simulink model "Sistema_Teste_Hugo_1"  (R2019a)
settings: Solver=ode23t  StartTime=0.0  StopTime=86400  MaxStep=6  RelTol=1e-3  EnableMultiTasking=on
InitFcn:
  | Dados_do_Sistema
undefined symbols (not defined in the file or in its folder): D1, Dados, Delta
libraries: powerlib x263, powerlib_meascontrol x79, dspsrcs4 x50
(part 1 of 5)
Description:
  | Copyright 2008-2014 The MathWorks, Inc.
settings Model: Creator=MathWorks  LastModifiedBy=hugo1
settings DataIOCC: LimitDataPoints=on  SaveFormat=Array  SignalLoggingSaveFormat=ModelDataLogs  SaveOutput=off  SaveTime=off  ReturnWorkspaceOutputs=off
settings OptimizationCC: ExpressionDepthLimit=2147483647  LifeSpan=inf
settings DebuggingCC: ReadBeforeWriteMsg=DisableAll  WriteAfterWriteMsg=DisableAll  WriteAfterReadMsg=DisableAll  UnderspecifiedInitializationDetection=Classic  MergeDetectMultiDrivingBlocksExec=none  SolverPrmCheckMsg=warning  ParameterPrecisionLossMsg=none  FcnCallInpInsideContextMsg=warning  UnconnectedInputMsg=none  UnconnectedOutputMsg=none  UnconnectedLineMsg=none  StateNameClashWarn=warning  SFUnexpectedBacktrackingDiag=warning  SFNoUnconditionalDefaultTransitionDiag=warning  SFExecutionAtInitializationDiag=none  ArithmeticOperatorsInVariantConditions=warning
settings HardwareCC: ProdBitPerPointer=32  ProdBitPerSizeT=32  ProdBitPerPtrDiffT=32  ProdLargestAtomicFloat=None  ProdIntDivRoundTo=Undefined  ProdEndianess=Unspecified  ProdWordSize=32  ProdHWDeviceType=32-bit Generic
settings ModelReferenceCC: PropagateSignalLabelsOutOfModel=off
settings SFSimCC: SimUseLocalCustomCode=off
settings RTWCC: RTWUseLocalCustomCode=off
settings CodeAppCC: StateflowObjectComments=on
settings GRTTargetCC: TargetLangStandard=C89/C90 (ANSI)  GeneratePreprocessorConditionals=Disable all  CombineOutputUpdateFcns=off  GRTInterface=on
settings ConfigComp: CovMetricSettings=dw  CovHtmlReporting=on  CovSaveCumulativeToWorkspaceVar=on  CovSaveSingleToWorkspaceVar=on  CovExternalEMLEnable=off  CovSFcnEnable=off
settings SimscapeCC: SimscapeNormalizeSystem=off

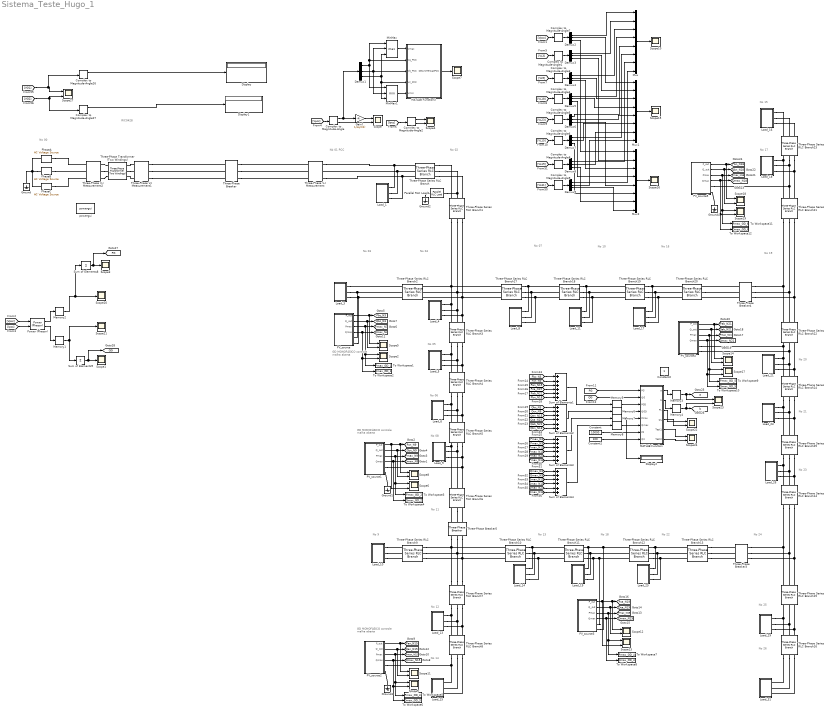
== system Sistema_Teste_Hugo_1 ==
  note: No 00
  note: RIC0428
  note: Nó 01 PCC
  note: No 02
  note: No 04
  note: No 03
  note: No 05
  note: No 06
  note: No 08
  note: No 11
  note: No 12
  note: No 14
  note: No 9
  note: No 13
  note: No 18
  note: No 22
  note: No 24
  note: No 25
  note: No 26
  note: No 20
  note: No 17
  note: No 15
  note: No 21
  note: No 23
  note: GD MONOFÁSICO
      | controle malha aberta
  note: GD MONOFÁSICO
      | controle malha aberta
  note: GD MONOFÁSICO
      | controle malha aberta
  note: No 07
  note: No 10
  note: No 16
  note: No 19
  Complex to Magnitude-Angle{,2,26..27} (4 alike) : ComplexToMagnitudeAngle
  Complex to Magnitude-Angle{1,3..9} (8 alike) : ComplexToMagnitudeAngle  Output=Magnitude
  Constant : Constant  Value=10000
  Constant1 : Constant  Value=100
  Constant2 : Constant
  Demux{1..9} (9 alike) : Demux  Outputs=3
  Display : Display
  Display1 : Display
  Display2 : Display
      settings: Decimation=3
  Gain1 : Gain  Gain=1/sqrt(2)
  Ground{,1..4} (5 alike) : powerlib/Elements/Ground  LConnTagsString=a
      settings: SourceProductName=Simscape Electrical
  Load_1 : Subsystem
  Load_10 : Subsystem
  Load_11 : Subsystem
  Load_13 : Subsystem
  Load_14 : Subsystem
  Load_15 : Subsystem
  Load_16 : Subsystem
  Load_17 : Subsystem
  Load_18 : Subsystem
  Load_19 : Subsystem
  Load_21 : Subsystem
  Load_23 : Subsystem
  Load_25 : Subsystem
  Load_26 : Subsystem
  Load_29 : Subsystem
  Load_3 : Subsystem
  Load_31 : Subsystem
  Load_4 : Subsystem
  Load_5 : Subsystem
  Load_6 : Subsystem
  Load_8 : Subsystem
  Load_9 : Subsystem
  MATLAB Function : MATLAB Function  TreatAsAtomicUnit=on
  MATLAB Function3 : MATLAB Function  TreatAsAtomicUnit=on
  Memory{1..8} (8 alike) : Memory
  MinMax : MinMax  Function=max  Inputs=3
  MinMax1 : MinMax  Inputs=3
  Mux : Mux  Inputs=8
  Mux1 : Mux  Inputs=8
  Mux2 : Mux  Inputs=8
  PV_source : Subsystem
  PV_source1 : Subsystem
  PV_source2 : Subsystem
  PV_source3 : Subsystem
  PV_source4 : Subsystem
  PV_source5 : Subsystem
  Parallel RLC Load1 : powerlib/Elements/Parallel RLC Load  LConnTagsString=a  RConnTagsString=__new0  NominalVoltage=127  NominalFrequency=60  ActivePower=100  InductivePower=40  CapacitivePower=0  Setx0=off  InitialVoltage=0  SetiL0=off  InitialCurrent=0  Measurements=None  LoadType=constant Z
      settings: AttributesFormatString=\n  SourceProductName=Simscape Electrical  SourceProductBaseCode=PS
  PhaseA : powerlib/Electrical Sources/AC Voltage Source  Amplitude=Dados.Tensao.va(1)  Phase=Dados.Tensao.va(2)  Frequency=Dados.Freq  SampleTime=0  Measurements=None  BusType=swing  Pref=10e3  Qref=0  Qmin=-inf  Qmax=+inf
      settings: SourceProductName=Simscape Electrical
  PhaseB : powerlib/Electrical Sources/AC Voltage Source  Amplitude=Dados.Tensao.vb(1)  Phase=Dados.Tensao.vb(2)  Frequency=Dados.Freq  SampleTime=0  Measurements=None  BusType=swing  Pref=10e3  Qref=0  Qmin=-inf  Qmax=+inf
      settings: SourceProductName=Simscape Electrical
  PhaseC : powerlib/Electrical Sources/AC Voltage Source  Amplitude=Dados.Tensao.vc(1)  Phase=Dados.Tensao.vc(2)  Frequency=Dados.Freq  SampleTime=0  Measurements=None  BusType=swing  Pref=10e3  Qref=0  Qmin=-inf  Qmax=+inf
      settings: SourceProductName=Simscape Electrical
  Power (Phasor) : powerlib_meascontrol/Measurements/Power (Phasor)
      settings: SourceProductName=Simscape Electrical  SourceProductBaseCode=PS
  Scope{,2,4..6,8..9,11..14,17..19,22..24,27} (18 alike) : Scope  NumInputPorts=2
  Scope{1,3,7,10,15..16,20..21} (8 alike) : Scope
  Sum of Elements{1..4} (4 alike) : Sum  Inputs=++++++
  Sum of Elements8 : Sum  Inputs=+
  Sum of Elements9 : Sum  Inputs=+
  Three-Phase Series RLC Branch : powerlib/Elements/Three-Phase Series RLC Branch  LConnTagsString=A|B|C  RConnTagsString=A|B|C  BranchType=RL  Resistance=Dados.Linha.Linha_01_02(1)  Inductance=Dados.Linha.Linha_01_02(2)  Capacitance=inf  Measurements=Branch currents
      settings: SourceProductName=Simscape Electrical
  Three-Phase Series RLC Branch1 : powerlib/Elements/Three-Phase Series RLC Branch  LConnTagsString=A|B|C  RConnTagsString=A|B|C  BranchType=RL  Resistance=Dados.Linha.Linha_02_04(1)  Inductance=Dados.Linha.Linha_02_04(2)  Capacitance=inf  Measurements=Branch currents
      settings: SourceProductName=Simscape Electrical
  Three-Phase Series RLC Branch10 : powerlib/Elements/Three-Phase Series RLC Branch  LConnTagsString=A|B|C  RConnTagsString=A|B|C  BranchType=RL  Resistance=Dados.Linha.Linha_11_13(1)  Inductance=Dados.Linha.Linha_11_13(2)  Capacitance=inf  Measurements=Branch currents
      settings: SourceProductName=Simscape Electrical
  Three-Phase Series RLC Branch11 : powerlib/Elements/Three-Phase Series RLC Branch  LConnTagsString=A|B|C  RConnTagsString=A|B|C  BranchType=RL  Resistance=Dados.Linha.Linha_13_18(1)  Inductance=Dados.Linha.Linha_13_18(2)  Capacitance=inf  Measurements=Branch currents
      settings: SourceProductName=Simscape Electrical
  Three-Phase Series RLC Branch12 : powerlib/Elements/Three-Phase Series RLC Branch  LConnTagsString=A|B|C  RConnTagsString=A|B|C  BranchType=RL  Resistance=Dados.Linha.Linha_18_22(1)  Inductance=Dados.Linha.Linha_18_22(2)  Capacitance=inf  Measurements=Branch currents
      settings: SourceProductName=Simscape Electrical
  Three-Phase Series RLC Branch13 : powerlib/Elements/Three-Phase Series RLC Branch  LConnTagsString=A|B|C  RConnTagsString=A|B|C  BranchType=RL  Resistance=Dados.Linha.Linha_22_24(1)  Inductance=Dados.Linha.Linha_22_24(2)  Capacitance=inf  Measurements=Branch currents
      settings: SourceProductName=Simscape Electrical
  Three-Phase Series RLC Branch14 : powerlib/Elements/Three-Phase Series RLC Branch  LConnTagsString=A|B|C  RConnTagsString=A|B|C  BranchType=RL  Resistance=Dados.Linha.Linha_24_23(1)  Inductance=Dados.Linha.Linha_24_23(2)  Capacitance=inf  Measurements=None
      settings: SourceProductName=Simscape Electrical
  Three-Phase Series RLC Branch15 : powerlib/Elements/Three-Phase Series RLC Branch  LConnTagsString=A|B|C  RConnTagsString=A|B|C  BranchType=RL  Resistance=Dados.Linha.Linha_24_25(1)  Inductance=Dados.Linha.Linha_24_25(2)  Capacitance=inf  Measurements=Branch currents
      settings: SourceProductName=Simscape Electrical
  Three-Phase Series RLC Branch16 : powerlib/Elements/Three-Phase Series RLC Branch  LConnTagsString=A|B|C  RConnTagsString=A|B|C  BranchType=RL  Resistance=Dados.Linha.Linha_25_26(1)  Inductance=Dados.Linha.Linha_25_26(2)  Capacitance=inf  Measurements=Branch currents
      settings: SourceProductName=Simscape Electrical
  Three-Phase Series RLC Branch17 : powerlib/Elements/Three-Phase Series RLC Branch  LConnTagsString=A|B|C  RConnTagsString=A|B|C  BranchType=RL  Resistance=Dados.Linha.Linha_07_04(1)  Inductance=Dados.Linha.Linha_07_04(2)  Capacitance=inf  Measurements=Branch currents
      settings: SourceProductName=Simscape Electrical
  Three-Phase Series RLC Branch18 : powerlib/Elements/Three-Phase Series RLC Branch  LConnTagsString=A|B|C  RConnTagsString=A|B|C  BranchType=RL  Resistance=Dados.Linha.Linha_10_07(1)  Inductance=Dados.Linha.Linha_10_07(2)  Capacitance=inf  Measurements=Branch currents
      settings: SourceProductName=Simscape Electrical
  Three-Phase Series RLC Branch19 : powerlib/Elements/Three-Phase Series RLC Branch  LConnTagsString=A|B|C  RConnTagsString=A|B|C  BranchType=RL  Resistance=Dados.Linha.Linha_16_10(1)  Inductance=Dados.Linha.Linha_16_10(2)  Capacitance=inf  Measurements=Branch currents
      settings: SourceProductName=Simscape Electrical
  Three-Phase Series RLC Branch2 : powerlib/Elements/Three-Phase Series RLC Branch  LConnTagsString=A|B|C  RConnTagsString=A|B|C  BranchType=RL  Resistance=Dados.Linha.Linha_04_03(1)  Inductance=Dados.Linha.Linha_04_03(2)  Capacitance=inf  Measurements=Branch currents
      settings: SourceProductName=Simscape Electrical
  Three-Phase Series RLC Branch20 : powerlib/Elements/Three-Phase Series RLC Branch  LConnTagsString=A|B|C  RConnTagsString=A|B|C  BranchType=RL  Resistance=Dados.Linha.Linha_19_16(1)  Inductance=Dados.Linha.Linha_19_16(2)  Capacitance=inf  Measurements=Branch currents
      settings: SourceProductName=Simscape Electrical
  Three-Phase Series RLC Branch21 : powerlib/Elements/Three-Phase Series RLC Branch  LConnTagsString=A|B|C  RConnTagsString=A|B|C  BranchType=RL  Resistance=Dados.Linha.Linha_19_17(1)  Inductance=Dados.Linha.Linha_19_17(2)  Capacitance=inf  Measurements=Branch currents
      settings: SourceProductName=Simscape Electrical
  Three-Phase Series RLC Branch22 : powerlib/Elements/Three-Phase Series RLC Branch  LConnTagsString=A|B|C  RConnTagsString=A|B|C  BranchType=RL  Resistance=Dados.Linha.Linha_20_19(1)  Inductance=Dados.Linha.Linha_20_19(2)  Capacitance=inf  Measurements=None
      settings: SourceProductName=Simscape Electrical
  Three-Phase Series RLC Branch23 : powerlib/Elements/Three-Phase Series RLC Branch  LConnTagsString=A|B|C  RConnTagsString=A|B|C  BranchType=RL  Resistance=Dados.Linha.Linha_17_15(1)  Inductance=Dados.Linha.Linha_17_15(2)  Capacitance=inf  Measurements=Branch currents
      settings: SourceProductName=Simscape Electrical
  Three-Phase Series RLC Branch24 : powerlib/Elements/Three-Phase Series RLC Branch  LConnTagsString=A|B|C  RConnTagsString=A|B|C  BranchType=RL  Resistance=Dados.Linha.Linha_21_20(1)  Inductance=Dados.Linha.Linha_21_20(2)  Capacitance=inf  Measurements=Branch currents
      settings: SourceProductName=Simscape Electrical
  Three-Phase Series RLC Branch25 : powerlib/Elements/Three-Phase Series RLC Branch  LConnTagsString=A|B|C  RConnTagsString=A|B|C  BranchType=RL  Resistance=Dados.Linha.Linha_23_21(1)  Inductance=Dados.Linha.Linha_23_21(2)  Capacitance=inf  Measurements=Branch currents
      settings: SourceProductName=Simscape Electrical
  Three-Phase Series RLC Branch3 : powerlib/Elements/Three-Phase Series RLC Branch  LConnTagsString=A|B|C  RConnTagsString=A|B|C  BranchType=RL  Resistance=Dados.Linha.Linha_04_05(1)  Inductance=Dados.Linha.Linha_04_05(2)  Capacitance=inf  Measurements=None
      settings: SourceProductName=Simscape Electrical
  Three-Phase Series RLC Branch4 : powerlib/Elements/Three-Phase Series RLC Branch  LConnTagsString=A|B|C  RConnTagsString=A|B|C  BranchType=RL  Resistance=Dados.Linha.Linha_05_06(1)  Inductance=Dados.Linha.Linha_05_06(2)  Capacitance=inf  Measurements=Branch currents
      settings: SourceProductName=Simscape Electrical
  Three-Phase Series RLC Branch5 : powerlib/Elements/Three-Phase Series RLC Branch  LConnTagsString=A|B|C  RConnTagsString=A|B|C  BranchType=RL  Resistance=Dados.Linha.Linha_06_08(1)  Inductance=Dados.Linha.Linha_06_08(2)  Capacitance=inf  Measurements=Branch currents
      settings: SourceProductName=Simscape Electrical
  Three-Phase Series RLC Branch6 : powerlib/Elements/Three-Phase Series RLC Branch  LConnTagsString=A|B|C  RConnTagsString=A|B|C  BranchType=RL  Resistance=Dados.Linha.Linha_08_11(1)  Inductance=Dados.Linha.Linha_08_11(2)  Capacitance=inf  Measurements=Branch currents
      settings: SourceProductName=Simscape Electrical
  Three-Phase Series RLC Branch7 : powerlib/Elements/Three-Phase Series RLC Branch  LConnTagsString=A|B|C  RConnTagsString=A|B|C  BranchType=RL  Resistance=Dados.Linha.Linha_11_12(1)  Inductance=Dados.Linha.Linha_11_12(2)  Capacitance=inf  Measurements=Branch currents
      settings: SourceProductName=Simscape Electrical
  Three-Phase Series RLC Branch8 : powerlib/Elements/Three-Phase Series RLC Branch  LConnTagsString=A|B|C  RConnTagsString=A|B|C  BranchType=RL  Resistance=Dados.Linha.Linha_12_14(1)  Inductance=Dados.Linha.Linha_12_14(2)  Capacitance=inf  Measurements=Branch currents
      settings: SourceProductName=Simscape Electrical
  Three-Phase Series RLC Branch9 : powerlib/Elements/Three-Phase Series RLC Branch  LConnTagsString=A|B|C  RConnTagsString=A|B|C  BranchType=RL  Resistance=Dados.Linha.Linha_11_09(1)  Inductance=Dados.Linha.Linha_11_09(2)  Capacitance=inf  Measurements=None
      settings: SourceProductName=Simscape Electrical
  Three-Phase Transformer (Two Windings) : powerlib/Elements/Three-Phase Transformer (Two Windings)  Winding1Connection=Delta (D1)  Winding2Connection=Yg  CoreType=Three single-phase transformers  SetSaturation=off  Hysteresis=off  DataFile='hysteresis'  SetInitialFlux=off  Measurements=None  UNITS=pu  NominalPower=[ 75e3 , 60 ]  Winding1=[ 13.8e3 , 0.0076 , 0.0157 ]  Winding2=[ 220 , 0.0076 , 0.0157 ]  Rm=227  Lm=32.59  L0=0.5  Saturation=[ 0,0 ; 0.0024,1.2 ; 1.0,1.52 ]  InitialFluxes=[ 0.8 , -0.8 , 0.7 ]  BreakLoop=off  DiscreteSolver=Trapezoidal iterative  DataType=off  TransfoNumber=1
      settings: SourceProductName=Simscape Electrical
  Three-Phase V-I Measurement : powerlib/Measurements/Three-Phase V-I Measurement  VoltageMeasurement=phase-to-ground  SetLabelV=on  LabelV=Vpcc  Vpu=off  VpuLL=off  CurrentMeasurement=yes  SetLabelI=on  LabelI=Ipcc  Ipu=off  Pbase=100e6  Vbase=500e3  OutputType=Complex  PhasorSimulation=on  PSBequivalent=0
      settings: SourceProductName=Simscape Electrical
  Three-Phase V-I Measurement1 : powerlib/Measurements/Three-Phase V-I Measurement  VoltageMeasurement=phase-to-phase  SetLabelV=on  LabelV=VG2  Vpu=off  VpuLL=off  CurrentMeasurement=no  SetLabelI=off  LabelI=IG  Ipu=off  Pbase=100e6  Vbase=500e3  OutputType=Complex  PhasorSimulation=on  PSBequivalent=0
      settings: SourceProductName=Simscape Electrical
  Three-Phase V-I Measurement2 : powerlib/Measurements/Three-Phase V-I Measurement  VoltageMeasurement=phase-to-phase  SetLabelV=on  LabelV=VG1  Vpu=off  VpuLL=off  CurrentMeasurement=no  SetLabelI=off  LabelI=IG  Ipu=off  Pbase=100e6  Vbase=500e3  OutputType=Complex  PhasorSimulation=on  PSBequivalent=0
      settings: SourceProductName=Simscape Electrical
  Three-Phase Breaker : powerlib/Elements/Three-Phase Breaker  InitialState=closed  SwitchA=on  SwitchB=on  SwitchC=on  SwitchTimes=[200000]  External=off  BreakerResistance=0.01  SnubberResistance=1e6  SnubberCapacitance=inf  Measurements=None
      settings: SourceProductName=Simscape Electrical
  Three-Phase Breaker3 : powerlib/Elements/Three-Phase Breaker  InitialState=closed  SwitchA=on  SwitchB=on  SwitchC=on  SwitchTimes=[864000]  External=off  BreakerResistance=0.01  SnubberResistance=1e6  SnubberCapacitance=inf  Measurements=None
      settings: SourceProductName=Simscape Electrical
  Three-Phase Breaker4 : powerlib/Elements/Three-Phase Breaker  InitialState=closed  SwitchA=on  SwitchB=on  SwitchC=on  SwitchTimes=[864000]  External=off  BreakerResistance=0.01  SnubberResistance=1e6  SnubberCapacitance=inf  Measurements=None
      settings: SourceProductName=Simscape Electrical
  Three-Phase Breaker5 : powerlib/Elements/Three-Phase Breaker  InitialState=closed  SwitchA=on  SwitchB=on  SwitchC=on  SwitchTimes=[864000]  External=off  BreakerResistance=0.01  SnubberResistance=1e6  SnubberCapacitance=inf  Measurements=None
      settings: SourceProductName=Simscape Electrical
  To Workspace1 : ToWorkspace  VariableName=Pmax_GD_1  SampleTime=-1
      settings: Save2DSignal=2-D array (concatenate along first dimension)
  To Workspace10 : ToWorkspace  VariableName=Qmax_GD_5  SampleTime=-1
      settings: Save2DSignal=2-D array (concatenate along first dimension)
  To Workspace11 : ToWorkspace  VariableName=Pmax_GD_6  SampleTime=-1
      settings: Save2DSignal=2-D array (concatenate along first dimension)
  To Workspace12 : ToWorkspace  VariableName=Qmax_GD_6  SampleTime=-1
      settings: Save2DSignal=2-D array (concatenate along first dimension)
  To Workspace2 : ToWorkspace  VariableName=Qmax_GD_1  SampleTime=-1
      settings: Save2DSignal=2-D array (concatenate along first dimension)
  To Workspace3 : ToWorkspace  VariableName=Pmax_GD_2  SampleTime=-1
      settings: Save2DSignal=2-D array (concatenate along first dimension)
  To Workspace4 : ToWorkspace  VariableName=Qmax_GD_2  SampleTime=-1
      settings: Save2DSignal=2-D array (concatenate along first dimension)
  To Workspace5 : ToWorkspace  VariableName=Pmax_GD_3  SampleTime=-1
      settings: Save2DSignal=2-D array (concatenate along first dimension)
  To Workspace6 : ToWorkspace  VariableName=Qmax_GD_3  SampleTime=-1
      settings: Save2DSignal=2-D array (concatenate along first dimension)
  To Workspace7 : ToWorkspace  VariableName=Pmax_GD_4  SampleTime=-1
      settings: Save2DSignal=2-D array (concatenate along first dimension)
  To Workspace8 : ToWorkspace  VariableName=Qmax_GD_4  SampleTime=-1
      settings: Save2DSignal=2-D array (concatenate along first dimension)
  To Workspace9 : ToWorkspace  VariableName=Pmax_GD_5  SampleTime=-1
      settings: Save2DSignal=2-D array (concatenate along first dimension)
  powergui : powerlib/powergui  Priority=1  SimulationMode=Phasor  SampleTime=50e-6  frequency=60  Iterations=50  frequencyindice=60  Pbase=100e6  ErrMax=1e-4  UnitsV=kV  UnitsW=MW  buscounter=0  FunctionMessages=off  echomessages=off  EnableUseOfTLC=off  CurrentSourceSwitches=off  DisableSnubberDevices=off  DisableRonSwitches=off  DisableVfSwitches=off  DisplayEquations=off  AutomaticDiscreteSolvers=off  SolverType=Tustin  Interpol=off  ExternalGateDelay=off  methode=off  Ts=0  x0status=blocks  SPID=off  SwTol=0  HookPort=off  NonlinearTolerance=0  nMaxIteration=15  ContinueOnMaxIteration=off  RestoreLinks=warning  ResistiveCurrentMeasurement=off  Frange=[0:2:500]  Ylog=off  Xlog=on  ShowGrid=off  save=off  variable=ZData  structure=0  ZoomFFT=off  StartTime=0.0  cycles=1  DisplayStyle=1  fundamental=60  FreqAxis=off  MaxFrequency=1000  frequencyindicesteady=1  RmsSteady=1  display=off
      settings: SourceProductName=Simscape Electrical
  tag scope: PG=global, Pab_N21=global, Pan_N15=global, Pbc_N3=global, Pbn_N18=global, Pca_N19=global, Pcn_N9=global, Pmax_N15=global, Pmax_N18=global, Pmax_N19=global, Pmax_N21=global, Pmax_N3=global, Pmax_N9=global, QG=global, Qab_N21=global, Qan_N15=global, Qbc_N3=global, Qbn_N18=global, Qca_N19=global, Qcn_N9=global, Qmax_N15=global, Qmax_N18=global, Qmax_N19=global, Qmax_N21=global, Qmax_N3=global, Qmax_N9=global, a=global, b=global
  wires:
  [Vpcc] -> Power (Phasor)/1
  [Ipcc] -> Power (Phasor)/2
  [Vpcc] -> Complex to Magnitude-Angle/1
  Complex to Magnitude-Angle2/1 -> Scope4/1
  [Ipcc] -> Complex to Magnitude-Angle2/1
  Power (Phasor)/1 -> Memory2/1
  Memory2/1 -> Sum of Elements8/1, Scope20/1
  Memory1/1 -> Sum of Elements9/1, Scope21/1
  Power (Phasor)/2 -> Memory1/1
  Complex to Magnitude-Angle2/2 -> Scope4/2
  [Vpcc] -> Complex to Magnitude-Angle7/1
  [VL3] -> Complex to Magnitude-Angle1/1
  Complex to Magnitude-Angle1/1 -> Demux3/1
  [VL9] -> Complex to Magnitude-Angle3/1
  Complex to Magnitude-Angle3/1 -> Demux4/1
  [VL18] -> Complex to Magnitude-Angle4/1
  Complex to Magnitude-Angle4/1 -> Demux5/1
  [VL23] -> Complex to Magnitude-Angle5/1
  Complex to Magnitude-Angle5/1 -> Demux6/1
  [VL15] -> Complex to Magnitude-Angle6/1
  Complex to Magnitude-Angle6/1 -> Demux7/1
  Mux/1 -> Scope10/1
  Complex to Magnitude-Angle7/1 -> Demux2/1
  [VL19] -> Complex to Magnitude-Angle8/1
  Complex to Magnitude-Angle8/1 -> Demux8/1
  [VL31] -> Complex to Magnitude-Angle9/1
  Complex to Magnitude-Angle9/1 -> Demux9/1
  Mux1/1 -> Scope15/1
  Mux2/1 -> Scope16/1
  Demux2/1 -> Mux/1
  Demux3/1 -> Mux/2
  Demux4/1 -> Mux/3
  Demux5/1 -> Mux/4
  Demux6/1 -> Mux/5
  Demux7/1 -> Mux/6
  Demux8/1 -> Mux/7
  Demux9/1 -> Mux/8
  Demux2/2 -> Mux1/1
  Demux3/2 -> Mux1/2
  Demux4/2 -> Mux1/3
  Demux5/2 -> Mux1/4
  Demux6/2 -> Mux1/5
  Demux7/2 -> Mux1/6
  Demux8/2 -> Mux1/7
  Demux9/2 -> Mux1/8
  Demux2/3 -> Mux2/1
  Demux3/3 -> Mux2/2
  Demux4/3 -> Mux2/3
  Demux5/3 -> Mux2/4
  Demux6/3 -> Mux2/5
  Demux7/3 -> Mux2/6
  Demux8/3 -> Mux2/7
  Demux9/3 -> Mux2/8
  Sum of Elements9/1 -> [QG], Scope1/1
  Sum of Elements8/1 -> [PG], Scope3/1
  MinMax/1 -> MATLAB Function3/1(Vmax)
  Complex to Magnitude-Angle/1 -> Demux1/1, Gain1/1
  MinMax1/1 -> MATLAB Function3/5(Vmin)
  Demux1/1 -> MinMax1/1, MinMax/1, MATLAB Function3/2(Va_PCC)
  Demux1/3 -> MinMax1/3, MATLAB Function3/4(Vc_PCC), MinMax/3
  Demux1/2 -> MinMax1/2, MinMax/2, MATLAB Function3/3(Vb_PCC)
  MATLAB Function3/1(DesvioTensaoPCC) -> Scope7/1
  PV_source/3(Pmax) -> To Workspace1/1, Scope2/1, [Pmax_N3]
  PV_source/2(Q_out) -> Scope5/2, [Qbc_N3]
  PV_source/4(Qmax) -> To Workspace2/1, Scope2/2, [Qmax_N3]
  PV_source/1(P_out) -> Scope5/1, [Pbc_N3]
  PV_source1/1(P_out) -> Scope8/1, [Pcn_N9], Scope6/2
  PV_source1/2(Q_out) -> Scope8/2, [Qcn_N9]
  PV_source2/2(Q_out) -> Scope11/2, [Qan_N15]
  PV_source2/1(P_out) -> Scope11/1, [Pan_N15]
  PV_source3/1(P_out) -> Scope13/2, Scope12/1, [Pca_N19]
  PV_source3/2(Q_out) -> Scope12/2, [Qca_N19]
  PV_source4/2(Q_out) -> Scope14/2, [Qab_N21]
  PV_source4/1(P_out) -> Scope14/1, [Pab_N21]
  PV_source5/1(P_out) -> Scope18/1, [Pbn_N18]
  PV_source5/2(Q_out) -> Scope18/2, [Qbn_N18]
  Memory4/1 -> Scope23/2, [b]
  Memory3/1 -> Scope23/1, [a]
  [Pab_N21] -> Sum of Elements1/5
  [Pbn_N18] -> Sum of Elements1/6
  Constant/1 -> MATLAB Function/7(P0)
  [Pmax_N18] -> Sum of Elements3/6
  Constant1/1 -> MATLAB Function/8(Q0)
  Sum of Elements2/1 -> Memory6/1
  [Pbc_N3] -> Sum of Elements1/1
  [Qab_N21] -> Sum of Elements2/5
  [Pca_N19] -> Sum of Elements1/4
  Sum of Elements1/1 -> Memory5/1
  [Qmax_N19] -> Sum of Elements4/4
  Sum of Elements3/1 -> Memory7/1
  [Qmax_N15] -> Sum of Elements4/3
  [Qmax_N3] -> Sum of Elements4/1
  [Qcn_N9] -> Sum of Elements2/2
  [Qmax_N18] -> Sum of Elements4/6
  [Qbn_N18] -> Sum of Elements2/6
  [Pmax_N19] -> Sum of Elements3/4
  [Pmax_N9] -> Sum of Elements3/2
  [Pmax_N15] -> Sum of Elements3/3
  [Qan_N15] -> Sum of Elements2/3
  [Qmax_N9] -> Sum of Elements4/2
  [Qca_N19] -> Sum of Elements2/4
  [Pmax_N3] -> Sum of Elements3/1
  [PG] -> MATLAB Function/1(PG)
  [Pmax_N21] -> Sum of Elements3/5
  [QG] -> MATLAB Function/2(QG)
  [Pan_N15] -> Sum of Elements1/3
  [Qbc_N3] -> Sum of Elements2/1
  Sum of Elements4/1 -> Memory8/1
  [Pcn_N9] -> Sum of Elements1/2
  [Qmax_N21] -> Sum of Elements4/5
  Memory5/1 -> MATLAB Function/3(PGD)
  Memory6/1 -> MATLAB Function/4(QGD)
  Memory7/1 -> Display2/1, MATLAB Function/5(Pmax)
  Memory8/1 -> MATLAB Function/6(Qmax)
  MATLAB Function/3(PL) -> Scope22/1
  MATLAB Function/4(QL) -> Scope22/2
  MATLAB Function/5(Test1) -> Scope24/1
  MATLAB Function/6(Test2) -> Scope24/2
  [VG1] -> Complex to Magnitude-Angle26/1, Scope27/1
  [VG2] -> Complex to Magnitude-Angle27/1, Scope27/2
  Complex to Magnitude-Angle26/1 -> Display/1
  Complex to Magnitude-Angle27/1 -> Display1/1
  Complex to Magnitude-Angle/2 -> Scope/2
  Gain1/1 -> Scope/1
  PV_source1/4(Qmax) -> To Workspace4/1, [Qmax_N9]
  PV_source1/3(Pmax) -> To Workspace3/1, Scope6/1, [Pmax_N9]
  PV_source2/4(Qmax) -> To Workspace6/1, Scope9/2, [Qmax_N15]
  PV_source2/3(Pmax) -> To Workspace5/1, Scope9/1, [Pmax_N15]
  PV_source3/4(Qmax) -> To Workspace8/1, [Qmax_N19]
  PV_source3/3(Pmax) -> To Workspace7/1, Scope13/1, [Pmax_N19]
  PV_source4/4(Qmax) -> To Workspace10/1, Scope17/2, [Qmax_N21]
  PV_source4/3(Pmax) -> To Workspace9/1, Scope17/1, [Pmax_N21]
  PV_source5/4(Qmax) -> To Workspace12/1, Scope19/2, [Qmax_N18]
  PV_source5/3(Pmax) -> To Workspace11/1, Scope19/1, [Pmax_N18]
  MATLAB Function/1(a) -> Memory3/1
  MATLAB Function/2(b) -> Memory4/1
  connections:
  PhaseB/LConn1 -- Ground/LConn1 -- PhaseA/LConn1 -- PhaseC/LConn1
  Three-Phase V-I Measurement/RConn1 -- Load_1/RConn1 -- Three-Phase Series RLC Branch/LConn1
  Three-Phase V-I Measurement/RConn3 -- Load_1/RConn3 -- Three-Phase Series RLC Branch/LConn3
  Three-Phase Breaker/RConn1 -- Three-Phase V-I Measurement/LConn1
  Three-Phase Breaker/RConn2 -- Three-Phase V-I Measurement/LConn2
  Three-Phase Breaker/RConn3 -- Three-Phase V-I Measurement/LConn3
  Three-Phase Series RLC Branch/LConn2 -- Load_1/RConn2 -- Three-Phase V-I Measurement/RConn2
  Three-Phase V-I Measurement1/LConn1 -- Three-Phase Transformer (Two Windings)/RConn1
  Three-Phase V-I Measurement1/LConn3 -- Three-Phase Transformer (Two Windings)/RConn3
  Three-Phase Transformer (Two Windings)/RConn2 -- Three-Phase V-I Measurement1/LConn2
  Three-Phase V-I Measurement1/RConn2 -- Three-Phase Breaker/LConn2
  Three-Phase V-I Measurement1/RConn1 -- Three-Phase Breaker/LConn1
  Three-Phase V-I Measurement1/RConn3 -- Three-Phase Breaker/LConn3
  Three-Phase Series RLC Branch/RConn1 -- Three-Phase Series RLC Branch1/LConn1
  Three-Phase Series RLC Branch/RConn2 -- Parallel RLC Load1/LConn1 -- Three-Phase Series RLC Branch1/LConn2
  Three-Phase Series RLC Branch/RConn3 -- Three-Phase Series RLC Branch1/LConn3
  Three-Phase Series RLC Branch1/RConn2 -- Three-Phase Series RLC Branch17/RConn2 -- Three-Phase Series RLC Branch2/LConn2 -- Load_4/RConn2 -- Three-Phase Series RLC Branch3/LConn2
  Three-Phase Series RLC Branch3/RConn1 -- Load_5/RConn1 -- Three-Phase Series RLC Branch4/LConn1
  Three-Phase Series RLC Branch3/RConn2 -- Load_5/RConn2 -- Three-Phase Series RLC Branch4/LConn2
  Three-Phase Series RLC Branch3/RConn3 -- Load_5/RConn3 -- Three-Phase Series RLC Branch4/LConn3
  Three-Phase Series RLC Branch4/RConn1 -- Load_6/RConn1 -- Three-Phase Series RLC Branch5/LConn1
  Three-Phase Series RLC Branch4/RConn2 -- Load_6/RConn2 -- Three-Phase Series RLC Branch5/LConn2
  Three-Phase Series RLC Branch4/RConn3 -- Load_6/RConn3 -- Three-Phase Series RLC Branch5/LConn3
  Three-Phase Series RLC Branch5/RConn1 -- Three-Phase Series RLC Branch6/LConn1 -- Load_9/RConn1
  Three-Phase Series RLC Branch5/RConn2 -- Load_9/RConn2 -- Three-Phase Series RLC Branch6/LConn2
  Three-Phase Series RLC Branch5/RConn3 -- Load_9/RConn3 -- PV_source1/RConn1 -- Three-Phase Series RLC Branch6/LConn3
  Three-Phase Series RLC Branch7/LConn2 -- Three-Phase Series RLC Branch10/RConn2 -- Three-Phase Breaker5/LConn2 -- Three-Phase Series RLC Branch9/LConn2
  Three-Phase Series RLC Branch7/RConn1 -- Load_13/RConn1 -- Three-Phase Series RLC Branch8/LConn1
  Three-Phase Series RLC Branch7/RConn2 -- Load_13/RConn2 -- Three-Phase Series RLC Branch8/LConn2
  Three-Phase Series RLC Branch7/RConn3 -- Load_13/RConn3 -- Three-Phase Series RLC Branch8/LConn3
  Three-Phase Breaker3/RConn3 -- Three-Phase Series RLC Branch14/RConn3 -- Three-Phase Series RLC Branch15/LConn3
  Three-Phase Series RLC Branch25/RConn3 -- Load_26/RConn3 -- Three-Phase Series RLC Branch14/LConn3
  Three-Phase Series RLC Branch10/LConn1 -- Load_14/RConn1 -- Three-Phase Series RLC Branch11/RConn1
  Three-Phase Series RLC Branch11/LConn1 -- Load_19/RConn1 -- PV_source3/RConn2 -- Three-Phase Series RLC Branch12/RConn1
  Three-Phase Series RLC Branch12/LConn1 -- Load_25/RConn1 -- Three-Phase Series RLC Branch13/RConn1
  Three-Phase Series RLC Branch10/LConn2 -- Load_14/RConn2 -- Three-Phase Series RLC Branch11/RConn2
  Three-Phase Series RLC Branch11/LConn2 -- Load_19/RConn2 -- Three-Phase Series RLC Branch12/RConn2
  Three-Phase Series RLC Branch12/LConn2 -- Load_25/RConn2 -- Three-Phase Series RLC Branch13/RConn2
  Three-Phase Series RLC Branch10/LConn3 -- Load_14/RConn3 -- Three-Phase Series RLC Branch11/RConn3
  Three-Phase Series RLC Branch11/LConn3 -- Load_19/RConn3 -- PV_source3/RConn1 -- Three-Phase Series RLC Branch12/RConn3
  Three-Phase Series RLC Branch12/LConn3 -- Load_25/RConn3 -- Three-Phase Series RLC Branch13/RConn3
  Three-Phase Breaker3/RConn1 -- Three-Phase Series RLC Branch14/RConn1 -- Three-Phase Series RLC Branch15/LConn1
  Three-Phase Breaker3/RConn2 -- Three-Phase Series RLC Branch14/RConn2 -- Three-Phase Series RLC Branch15/LConn2
  Three-Phase Series RLC Branch16/LConn1 -- Load_29/RConn1 -- Three-Phase Series RLC Branch15/RConn1
  Three-Phase Series RLC Branch16/LConn2 -- Load_29/RConn2 -- Three-Phase Series RLC Branch15/RConn2
  Three-Phase Series RLC Branch16/LConn3 -- Load_29/RConn3 -- Three-Phase Series RLC Branch15/RConn3
  Three-Phase Series RLC Branch19/LConn1 -- Load_17/RConn1 -- Three-Phase Series RLC Branch20/RConn1
  Three-Phase Series RLC Branch18/LConn3 -- Load_11/RConn3 -- Three-Phase Series RLC Branch19/RConn3
  Three-Phase Series RLC Branch19/LConn3 -- Load_17/RConn3 -- Three-Phase Series RLC Branch20/RConn3
  Three-Phase Series RLC Branch18/LConn2 -- Load_11/RConn2 -- Three-Phase Series RLC Branch19/RConn2
  Three-Phase Series RLC Branch17/LConn3 -- Three-Phase Series RLC Branch18/RConn3 -- Load_8/RConn3
  Three-Phase Series RLC Branch17/LConn1 -- Three-Phase Series RLC Branch18/RConn1 -- Load_8/RConn1
  Three-Phase Series RLC Branch18/LConn1 -- Load_11/RConn1 -- Three-Phase Series RLC Branch19/RConn1
  Three-Phase Series RLC Branch17/LConn2 -- Three-Phase Series RLC Branch18/RConn2 -- Load_8/RConn2
  Three-Phase Series RLC Branch19/LConn2 -- Load_17/RConn2 -- Three-Phase Series RLC Branch20/RConn2
  Three-Phase Breaker4/RConn1 -- Three-Phase Series RLC Branch21/RConn1 -- Three-Phase Series RLC Branch22/LConn1
  Three-Phase Breaker4/RConn2 -- Three-Phase Series RLC Branch21/RConn2 -- Three-Phase Series RLC Branch22/LConn2
  Three-Phase Breaker4/RConn3 -- Three-Phase Series RLC Branch21/RConn3 -- Three-Phase Series RLC Branch22/LConn3
  Three-Phase Series RLC Branch23/RConn3 -- Three-Phase Series RLC Branch21/LConn3 -- Load_18/RConn3
  Three-Phase Series RLC Branch23/RConn2 -- PV_source5/RConn1 -- Three-Phase Series RLC Branch21/LConn2 -- Load_18/RConn2
  Three-Phase Series RLC Branch23/RConn1 -- Three-Phase Series RLC Branch21/LConn1 -- Load_18/RConn1
  Three-Phase Series RLC Branch24/RConn2 -- Load_23/RConn2 -- Three-Phase Series RLC Branch25/LConn2
  Three-Phase Series RLC Branch24/RConn1 -- Load_23/RConn1 -- Three-Phase Series RLC Branch25/LConn1
  Three-Phase Series RLC Branch24/RConn3 -- Load_23/RConn3 -- Three-Phase Series RLC Branch25/LConn3
  Three-Phase Series RLC Branch24/LConn3 -- Load_21/RConn3 -- Three-Phase Series RLC Branch22/RConn3
  Three-Phase Series RLC Branch24/LConn2 -- Load_21/RConn2 -- Three-Phase Series RLC Branch22/RConn2 -- PV_source4/RConn2
  Three-Phase Series RLC Branch24/LConn1 -- Load_21/RConn1 -- PV_source4/RConn1 -- Three-Phase Series RLC Branch22/RConn1
  Three-Phase Series RLC Branch25/RConn1 -- Load_26/RConn1 -- Three-Phase Series RLC Branch14/LConn1
  Three-Phase Series RLC Branch25/RConn2 -- Load_26/RConn2 -- Three-Phase Series RLC Branch14/LConn2
  Three-Phase Series RLC Branch13/LConn1 -- Three-Phase Breaker3/LConn1
  Three-Phase Series RLC Branch13/LConn2 -- Three-Phase Breaker3/LConn2
  Three-Phase Series RLC Branch13/LConn3 -- Three-Phase Breaker3/LConn3
  Three-Phase Breaker4/LConn1 -- Three-Phase Series RLC Branch20/LConn1
  Three-Phase Series RLC Branch20/LConn2 -- Three-Phase Breaker4/LConn2
  Three-Phase Breaker4/LConn3 -- Three-Phase Series RLC Branch20/LConn3
  Three-Phase Breaker5/RConn1 -- Three-Phase Series RLC Branch6/RConn1
  Three-Phase Series RLC Branch6/RConn2 -- Three-Phase Breaker5/RConn2
  Three-Phase Breaker5/RConn3 -- Three-Phase Series RLC Branch6/RConn3
  Load_3/RConn3 -- Three-Phase Series RLC Branch2/RConn3 -- PV_source/RConn2
  Load_3/RConn2 -- PV_source/RConn1 -- Three-Phase Series RLC Branch2/RConn2
  Parallel RLC Load1/RConn1 -- Ground2/LConn1
  Load_10/RConn1 -- Three-Phase Series RLC Branch9/RConn1
  Load_10/RConn2 -- Three-Phase Series RLC Branch9/RConn2
  Load_10/RConn3 -- Three-Phase Series RLC Branch9/RConn3
  Load_16/RConn3 -- Three-Phase Series RLC Branch23/LConn3
  Load_16/RConn2 -- Three-Phase Series RLC Branch23/LConn2
  Load_16/RConn1 -- Three-Phase Series RLC Branch23/LConn1
  Three-Phase Series RLC Branch16/RConn1 -- Load_31/RConn1
  Three-Phase Series RLC Branch16/RConn2 -- Load_31/RConn2
  Three-Phase Series RLC Branch16/RConn3 -- Load_31/RConn3
  Three-Phase Series RLC Branch7/LConn1 -- Three-Phase Series RLC Branch10/RConn1 -- Three-Phase Breaker5/LConn1 -- Three-Phase Series RLC Branch9/LConn1
  Three-Phase Series RLC Branch7/LConn3 -- Three-Phase Series RLC Branch10/RConn3 -- Three-Phase Breaker5/LConn3 -- Three-Phase Series RLC Branch9/LConn3
  Three-Phase Series RLC Branch8/RConn1 -- PV_source2/RConn1 -- Load_15/RConn1
  Three-Phase Series RLC Branch8/RConn2 -- Load_15/RConn2
  Three-Phase Series RLC Branch8/RConn3 -- Load_15/RConn3
  Three-Phase Series RLC Branch1/RConn3 -- Three-Phase Series RLC Branch17/RConn3 -- Load_4/RConn3 -- Three-Phase Series RLC Branch3/LConn3 -- Three-Phase Series RLC Branch2/LConn3
  Three-Phase Series RLC Branch1/RConn1 -- Three-Phase Series RLC Branch17/RConn1 -- Load_4/RConn1 -- Three-Phase Series RLC Branch3/LConn1 -- Three-Phase Series RLC Branch2/LConn1
  Load_3/RConn1 -- Three-Phase Series RLC Branch2/RConn1
  Ground1/LConn1 -- PV_source1/RConn2
  Ground3/LConn1 -- PV_source2/RConn2
  Ground4/LConn1 -- PV_source5/RConn2
  Three-Phase V-I Measurement2/RConn2 -- Three-Phase Transformer (Two Windings)/LConn2
  Three-Phase V-I Measurement2/RConn1 -- Three-Phase Transformer (Two Windings)/LConn1
  Three-Phase V-I Measurement2/RConn3 -- Three-Phase Transformer (Two Windings)/LConn3
  PhaseA/RConn1 -- Three-Phase V-I Measurement2/LConn1
  PhaseB/RConn1 -- Three-Phase V-I Measurement2/LConn2
  PhaseC/RConn1 -- Three-Phase V-I Measurement2/LConn3

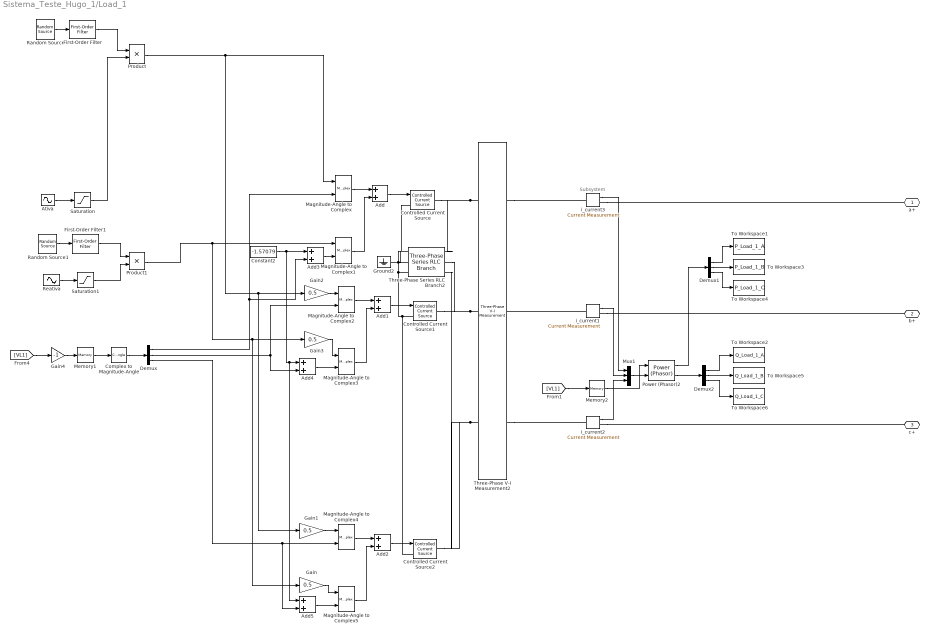
== system Sistema_Teste_Hugo_1/Load_1 ==
  note: Subsystem
  Add{,1..5} (6 alike) : Sum
  Ativa : Sin  Amplitude=10  Frequency=6.9e-5  Phase=-3.14  SampleTime=0
  Complex to Magnitude-Angle : ComplexToMagnitudeAngle  Output=Angle
  Constant2 : Constant  Value=-1.57079
  Controlled Current Source : powerlib/Electrical Sources/Controlled Current Source  Initialize=off  Source_Type=AC  Amplitude=0  Phase=0  Frequency=0  Measurements=None
      settings: SourceProductName=Simscape Electrical
  Controlled Current Source1 : powerlib/Electrical Sources/Controlled Current Source  Initialize=off  Source_Type=AC  Amplitude=0  Phase=0  Frequency=0  Measurements=None
      settings: SourceProductName=Simscape Electrical
  Controlled Current Source2 : powerlib/Electrical Sources/Controlled Current Source  Initialize=off  Source_Type=AC  Amplitude=0  Phase=0  Frequency=0  Measurements=None
      settings: SourceProductName=Simscape Electrical
  Demux : Demux  Outputs=3
  Demux1 : Demux  Outputs=3
  Demux2 : Demux  Outputs=3
  First-Order Filter : powerlib_meascontrol/Filters/First-Order Filter  FilterType=Lowpass  Tc=200  Ts=0  Initialize=on  Vac_Init=[0, 0, Dados.Freq]  Vdc_Init=1  PlotResponse=off  FreqRange="[0,  200,  1]"
      settings: SourceProductName=Simscape Electrical
  First-Order Filter1 : powerlib_meascontrol/Filters/First-Order Filter  FilterType=Lowpass  Tc=400  Ts=0  Initialize=on  Vac_Init=[0, 0, Dados.Freq]  Vdc_Init=1  PlotResponse=off  FreqRange="[0,  200,  1]"
      settings: SourceProductName=Simscape Electrical
  Gain{,1..3} (4 alike) : Gain  Gain=0.5
  Gain4 : Gain  Gain=-1
  Ground2 : powerlib/Elements/Ground  LConnTagsString=a
      settings: SourceProductName=Simscape Electrical
  Magnitude-Angle to Complex{,1..5} (6 alike) : MagnitudeAngleToComplex
  Memory1 : Memory
  Memory2 : Memory
  Mux1 : Mux  Inputs=3
  Power (Phasor)2 : powerlib_meascontrol/Measurements/Power (Phasor)
      settings: SourceProductName=Simscape Electrical  SourceProductBaseCode=PS
  Product : Product
  Product1 : Product
  Random Source : dspsrcs4/Random Source  SrcType=Uniform  NormMethod=Ziggurat  CltLength=12  MinVal=0.6  MaxVal=1  MeanVal=0  VarVal=1  RepMode=Repeatable  rawSeed=1  IsInherit=off  SampMode=Discrete  SampTime=200  SampFrame=1  DataType=Single  OutComplex=Real  OutputFrames=on
  Random Source1 : dspsrcs4/Random Source  SrcType=Uniform  NormMethod=Ziggurat  CltLength=12  MinVal=0.8  MaxVal=1.05  MeanVal=0  VarVal=1  RepMode=Repeatable  rawSeed=1  IsInherit=off  SampMode=Discrete  SampTime=400  SampFrame=1  DataType=Single  OutComplex=Real  OutputFrames=on
  Reativa : Sin  Amplitude=4  Frequency=6.9e-5  Phase=-3.14  SampleTime=0
  Saturation : Saturate  UpperLimit=36  LowerLimit=5
  Saturation1 : Saturate  UpperLimit=10  LowerLimit=3
  Three-Phase Series RLC Branch2 : powerlib/Elements/Three-Phase Series RLC Branch  LConnTagsString=A|B|C  RConnTagsString=A|B|C  BranchType=RC  Resistance=0.0001  Inductance=5.46e-6  Capacitance=1e-9  Measurements=None
      settings: SourceProductName=Simscape Electrical
  Three-Phase V-I Measurement2 : powerlib/Measurements/Three-Phase V-I Measurement  VoltageMeasurement=phase-to-ground  SetLabelV=on  LabelV=VL1  Vpu=off  VpuLL=off  CurrentMeasurement=no  SetLabelI=on  LabelI=IL1  Ipu=off  Pbase=100e6  Vbase=500e3  OutputType=Complex  PhasorSimulation=on  PSBequivalent=0
      settings: SourceProductName=Simscape Electrical
  To Workspace1 : ToWorkspace  VariableName=P_Load_1_A  SampleTime=-1
  To Workspace2 : ToWorkspace  VariableName=Q_Load_1_A  SampleTime=-1
  To Workspace3 : ToWorkspace  VariableName=P_Load_1_B  SampleTime=-1
  To Workspace4 : ToWorkspace  VariableName=P_Load_1_C  SampleTime=-1
  To Workspace5 : ToWorkspace  VariableName=Q_Load_1_B  SampleTime=-1
  To Workspace6 : ToWorkspace  VariableName=Q_Load_1_C  SampleTime=-1
  i_current1 : powerlib/Measurements/Current Measurement  PhasorSimulation=on  OutputType=Complex  PSBequivalent=0
      settings: SourceProductName=Simscape Electrical
  i_current2 : powerlib/Measurements/Current Measurement  PhasorSimulation=on  OutputType=Complex  PSBequivalent=0
      settings: SourceProductName=Simscape Electrical
  i_current3 : powerlib/Measurements/Current Measurement  PhasorSimulation=on  OutputType=Complex  PSBequivalent=0
      settings: SourceProductName=Simscape Electrical
  a+ : PMIOPort  Side=Right
  b+ : PMIOPort  Port=2  Side=Right
  c+ : PMIOPort  Port=3  Side=Right
  wires:
  Ativa/1 -> Saturation/1
  Saturation/1 -> Product/2
  Random Source/1 -> First-Order Filter/1
  First-Order Filter/1 -> Product/1
  Reativa/1 -> Saturation1/1
  First-Order Filter1/1 -> Product1/1
  Random Source1/1 -> First-Order Filter1/1
  Saturation1/1 -> Product1/2
  Add/1 -> Controlled Current Source/1
  Magnitude-Angle to Complex/1 -> Add/1
  Magnitude-Angle to Complex1/1 -> Add/2
  Add1/1 -> Controlled Current Source1/1
  Magnitude-Angle to Complex2/1 -> Add1/1
  Magnitude-Angle to Complex3/1 -> Add1/2
  Add2/1 -> Controlled Current Source2/1
  Magnitude-Angle to Complex4/1 -> Add2/1
  Magnitude-Angle to Complex5/1 -> Add2/2
  Complex to Magnitude-Angle/1 -> Demux/1
  Demux/1 -> Magnitude-Angle to Complex/2, Add3/2
  Constant2/1 -> Add5/1, Add4/1, Add3/1
  Add3/1 -> Magnitude-Angle to Complex1/2
  Add4/1 -> Magnitude-Angle to Complex3/2
  Demux/3 -> Magnitude-Angle to Complex4/2, Add5/2
  Add5/1 -> Magnitude-Angle to Complex5/2
  [VL1] -> Gain4/1
  Memory1/1 -> Complex to Magnitude-Angle/1
  Gain1/1 -> Magnitude-Angle to Complex4/1
  Gain/1 -> Magnitude-Angle to Complex5/1
  Product/1 -> Magnitude-Angle to Complex/1, Gain2/1, Gain1/1
  Product1/1 -> Magnitude-Angle to Complex1/1, Gain3/1, Gain/1
  Gain2/1 -> Magnitude-Angle to Complex2/1
  Gain3/1 -> Magnitude-Angle to Complex3/1
  Gain4/1 -> Memory1/1
  Demux/2 -> Add4/2, Magnitude-Angle to Complex2/2
  [VL1] -> Memory2/1
  Demux1/1 -> To Workspace1/1
  Demux1/2 -> To Workspace3/1
  i_current2/1 -> Mux1/3
  i_current3/1 -> Mux1/1
  i_current1/1 -> Mux1/2
  Mux1/1 -> Power (Phasor)2/2
  Demux1/3 -> To Workspace4/1
  Power (Phasor)2/1 -> Demux1/1
  Power (Phasor)2/2 -> Demux2/1
  Demux2/2 -> To Workspace5/1
  Demux2/1 -> To Workspace2/1
  Demux2/3 -> To Workspace6/1
  Memory2/1 -> Power (Phasor)2/1
  connections:
  Three-Phase V-I Measurement2/RConn1 -- Three-Phase Series RLC Branch2/LConn1 -- Controlled Current Source/RConn1
  Three-Phase V-I Measurement2/RConn2 -- Controlled Current Source1/RConn1 -- Three-Phase Series RLC Branch2/LConn2
  Three-Phase V-I Measurement2/RConn3 -- Controlled Current Source2/RConn1 -- Three-Phase Series RLC Branch2/LConn3
  Controlled Current Source1/LConn1 -- Three-Phase Series RLC Branch2/RConn3 -- Three-Phase Series RLC Branch2/RConn1 -- Controlled Current Source/LConn1 -- Three-Phase Series RLC Branch2/RConn2 -- Ground2/LConn1 -- Controlled Current Source2/LConn1
  i_current3/RConn1 -- a+/RConn1
  i_current1/LConn1 -- Three-Phase V-I Measurement2/LConn2
  i_current1/RConn1 -- b+/RConn1
  i_current2/RConn1 -- c+/RConn1
  Three-Phase V-I Measurement2/LConn3 -- i_current2/LConn1
  Three-Phase V-I Measurement2/LConn1 -- i_current3/LConn1

== system Sistema_Teste_Hugo_1/Load_10 ==
  note: Subsystem
  Add{,1..5} (6 alike) : Sum
  Ativa : Sin  Amplitude=8  Frequency=6.9e-5  Phase=-3.14  SampleTime=0
  Complex to Magnitude-Angle : ComplexToMagnitudeAngle  Output=Angle
  Constant2 : Constant  Value=-1.57079
  Controlled Current Source : powerlib/Electrical Sources/Controlled Current Source  Initialize=off  Source_Type=AC  Amplitude=0  Phase=0  Frequency=0  Measurements=None
      settings: SourceProductName=Simscape Electrical
  Controlled Current Source1 : powerlib/Electrical Sources/Controlled Current Source  Initialize=off  Source_Type=AC  Amplitude=0  Phase=0  Frequency=0  Measurements=None
      settings: SourceProductName=Simscape Electrical
  Controlled Current Source2 : powerlib/Electrical Sources/Controlled Current Source  Initialize=off  Source_Type=AC  Amplitude=0  Phase=0  Frequency=0  Measurements=None
      settings: SourceProductName=Simscape Electrical
  Demux : Demux  Outputs=3
  Demux1 : Demux  Outputs=3
  Demux2 : Demux  Outputs=3
  First-Order Filter : powerlib_meascontrol/Filters/First-Order Filter  FilterType=Lowpass  Tc=200  Ts=0  Initialize=on  Vac_Init=[0, 0, 60]  Vdc_Init=1  PlotResponse=off  FreqRange="[0,  200,  1]"
      settings: SourceProductName=Simscape Electrical
  First-Order Filter1 : powerlib_meascontrol/Filters/First-Order Filter  FilterType=Lowpass  Tc=400  Ts=0  Initialize=on  Vac_Init=[0, 0, 60]  Vdc_Init=1  PlotResponse=off  FreqRange="[0,  200,  1]"
      settings: SourceProductName=Simscape Electrical
  Gain4 : Gain  Gain=-1
  Ground2 : powerlib/Elements/Ground  LConnTagsString=a
      settings: SourceProductName=Simscape Electrical
  Magnitude-Angle to Complex{,1..5} (6 alike) : MagnitudeAngleToComplex
  Memory1 : Memory
  Memory2 : Memory
  Mux1 : Mux  Inputs=3
  Power (Phasor)2 : powerlib_meascontrol/Measurements/Power (Phasor)
      settings: SourceProductName=Simscape Electrical  SourceProductBaseCode=PS
  Product : Product
  Product1 : Product
  Random Source : dspsrcs4/Random Source  SrcType=Uniform  NormMethod=Ziggurat  CltLength=12  MinVal=0.7  MaxVal=1  MeanVal=0  VarVal=1  RepMode=Repeatable  rawSeed=1  IsInherit=off  SampMode=Discrete  SampTime=200  SampFrame=1  DataType=Single  OutComplex=Real  OutputFrames=on
  Random Source1 : dspsrcs4/Random Source  SrcType=Uniform  NormMethod=Ziggurat  CltLength=12  MinVal=0.65  MaxVal=1  MeanVal=0  VarVal=1  RepMode=Repeatable  rawSeed=1  IsInherit=off  SampMode=Discrete  SampTime=400  SampFrame=1  DataType=Single  OutComplex=Real  OutputFrames=on
  Reativa : Sin  Amplitude=3  Frequency=6.9e-5  Phase=-3.14  SampleTime=0
  Saturation : Saturate  UpperLimit=36  LowerLimit=4
  Saturation1 : Saturate  UpperLimit=10  LowerLimit=2.5
  Three-Phase Series RLC Branch2 : powerlib/Elements/Three-Phase Series RLC Branch  LConnTagsString=A|B|C  RConnTagsString=A|B|C  BranchType=RC  Resistance=0.0001  Inductance=5.46e-6  Capacitance=1e-9  Measurements=None
      settings: SourceProductName=Simscape Electrical
  Three-Phase V-I Measurement2 : powerlib/Measurements/Three-Phase V-I Measurement  VoltageMeasurement=phase-to-ground  SetLabelV=on  LabelV=VL10  Vpu=off  VpuLL=off  CurrentMeasurement=no  SetLabelI=on  LabelI=IL10  Ipu=off  Pbase=100e6  Vbase=500e3  OutputType=Complex  PhasorSimulation=on  PSBequivalent=0
      settings: SourceProductName=Simscape Electrical
  To Workspace1 : ToWorkspace  VariableName=P_Load_10_A  SampleTime=-1
  To Workspace2 : ToWorkspace  VariableName=Q_Load_10_A  SampleTime=-1
  To Workspace3 : ToWorkspace  VariableName=P_Load_10_B  SampleTime=-1
  To Workspace4 : ToWorkspace  VariableName=P_Load_10_C  SampleTime=-1
  To Workspace5 : ToWorkspace  VariableName=Q_Load_10_B  SampleTime=-1
  To Workspace6 : ToWorkspace  VariableName=Q_Load_10_C  SampleTime=-1
  i_current1 : powerlib/Measurements/Current Measurement  PhasorSimulation=on  OutputType=Complex  PSBequivalent=0
      settings: SourceProductName=Simscape Electrical
  i_current2 : powerlib/Measurements/Current Measurement  PhasorSimulation=on  OutputType=Complex  PSBequivalent=0
      settings: SourceProductName=Simscape Electrical
  i_current3 : powerlib/Measurements/Current Measurement  PhasorSimulation=on  OutputType=Complex  PSBequivalent=0
      settings: SourceProductName=Simscape Electrical
  a+ : PMIOPort  Side=Right
  b+ : PMIOPort  Port=2  Side=Right
  c+ : PMIOPort  Port=3  Side=Right
  wires:
  Ativa/1 -> Saturation/1
  Saturation/1 -> Product/2
  Random Source/1 -> First-Order Filter/1
  First-Order Filter/1 -> Product/1
  Reativa/1 -> Saturation1/1
  First-Order Filter1/1 -> Product1/1
  Random Source1/1 -> First-Order Filter1/1
  Saturation1/1 -> Product1/2
  Add/1 -> Controlled Current Source/1
  Magnitude-Angle to Complex/1 -> Add/1
  Magnitude-Angle to Complex1/1 -> Add/2
  Add1/1 -> Controlled Current Source1/1
  Magnitude-Angle to Complex2/1 -> Add1/1
  Magnitude-Angle to Complex3/1 -> Add1/2
  Add2/1 -> Controlled Current Source2/1
  Magnitude-Angle to Complex4/1 -> Add2/1
  Magnitude-Angle to Complex5/1 -> Add2/2
  Complex to Magnitude-Angle/1 -> Demux/1
  Demux/1 -> Magnitude-Angle to Complex/2, Add3/2
  Constant2/1 -> Add5/1, Add4/1, Add3/1
  Add3/1 -> Magnitude-Angle to Complex1/2
  Demux/2 -> Add4/2, Magnitude-Angle to Complex2/2
  Add4/1 -> Magnitude-Angle to Complex3/2
  Demux/3 -> Magnitude-Angle to Complex4/2, Add5/2
  Add5/1 -> Magnitude-Angle to Complex5/2
  [VL10] -> Gain4/1
  Memory1/1 -> Complex to Magnitude-Angle/1
  Product/1 -> Magnitude-Angle to Complex/1, Magnitude-Angle to Complex2/1, Magnitude-Angle to Complex4/1
  Product1/1 -> Magnitude-Angle to Complex1/1, Magnitude-Angle to Complex3/1, Magnitude-Angle to Complex5/1
  Gain4/1 -> Memory1/1
  Demux2/2 -> To Workspace5/1
  Mux1/1 -> Power (Phasor)2/2
  i_current2/1 -> Mux1/3
  i_current1/1 -> Mux1/2
  Demux2/1 -> To Workspace2/1
  Demux1/2 -> To Workspace3/1
  Demux2/3 -> To Workspace6/1
  Demux1/3 -> To Workspace4/1
  Demux1/1 -> To Workspace1/1
  [VL10] -> Memory2/1
  Power (Phasor)2/1 -> Demux1/1
  i_current3/1 -> Mux1/1
  Power (Phasor)2/2 -> Demux2/1
  Memory2/1 -> Power (Phasor)2/1
  connections:
  Three-Phase V-I Measurement2/RConn1 -- Controlled Current Source/RConn1 -- Three-Phase Series RLC Branch2/LConn1
  Three-Phase V-I Measurement2/RConn2 -- Controlled Current Source1/RConn1 -- Three-Phase Series RLC Branch2/LConn2
  Three-Phase V-I Measurement2/RConn3 -- Controlled Current Source2/RConn1 -- Three-Phase Series RLC Branch2/LConn3
  Controlled Current Source1/LConn1 -- Three-Phase Series RLC Branch2/RConn3 -- Three-Phase Series RLC Branch2/RConn1 -- Controlled Current Source/LConn1 -- Three-Phase Series RLC Branch2/RConn2 -- Ground2/LConn1 -- Controlled Current Source2/LConn1
  c+/RConn1 -- i_current2/RConn1
  Three-Phase V-I Measurement2/LConn3 -- i_current2/LConn1
  a+/RConn1 -- i_current3/RConn1
  Three-Phase V-I Measurement2/LConn2 -- i_current1/LConn1
  b+/RConn1 -- i_current1/RConn1
  Three-Phase V-I Measurement2/LConn1 -- i_current3/LConn1
